simulink model "Problem5"  (R2022a)
settings: Solver=VariableStepAuto  StartTime=0.0  StopTime=t_final  MaxStep=max_step_size  RelTol=1e-3
values from neighbouring files (symbols this model uses):
  k_i_v = k_p_v^2/4    (= 0.25)    [Problem5Part2.m]    (also in Problem5Try1.m; Problem5part15.m; Problem6.m)
  k_p_v = 1    [Problem5Part2.m]    (also in Problem5Try1.m; Problem5part15.m; Problem6.m)
  k_p_y = 4/l_r    (= 2.35294117647)    [Problem5Part2.m]    (also in Problem5Try1.m; Problem5part15.m; Problem6.m)
  l_r = 1.7    [Problem2.m]    (also in Problem2Try2.m; Problem3Try1.m; Problem5Part2.m; Problem5Try1.m)
  psi_initial = psi_sweep(i)    [Problem3Try1.m]    (also in Problem5Part2.m = 0.1; Problem5Try1.m = psi_sweep(j); Problem5part15.m = 0.523598775598; Problem6.m = 0.1)
  v_initial = 0    [Problem5Part2.m]    (also in Problem5Try1.m = v_sweep(i); Problem5part15.m; Problem6.m)
  v_target = 15.6464    [Problem5Part2.m]    (also in Problem5Try1.m; Problem5part15.m; Problem6.m = 20)
  y_initial = 10^(y_sweep(j))    [Problem3Try1.m]    (also in Problem5Part2.m = 0.1; Problem5Try1.m = 10^(log_y_sweep(k)); Problem5part15.m = 0.1; Problem6.m = 0.1)
  y_target = 0    [Problem5Part2.m]    (also in Problem5Try1.m; Problem5part15.m; Problem6.m)
settings Model: Creator=Lawrence  LastModifiedBy=Lawrence

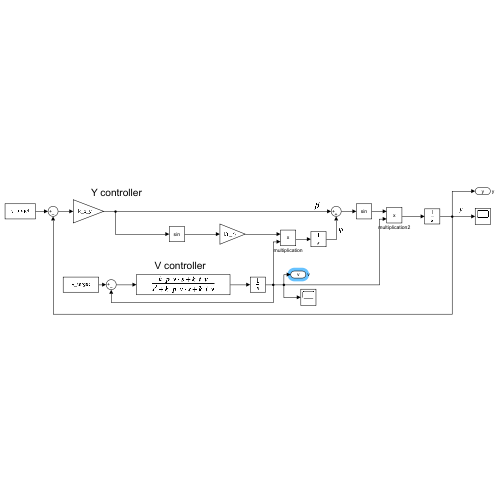
[thumbnail: Simulink's stored preview of the top-level diagram]
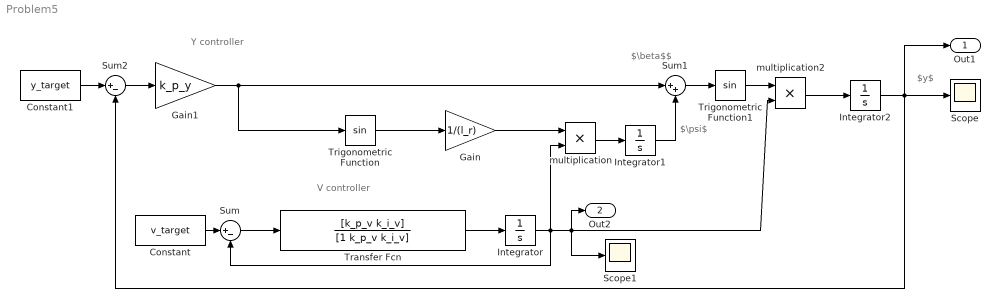
== system Problem5 ==
  note: $y$
  note: $\psi$
  note: $\beta$$
  note: V controller
  note: Y controller
  Constant : Constant  Value=v_target
  Constant1 : Constant  Value=y_target
  Gain : Gain  Gain=1/(l_r)
  Gain1 : Gain  Gain=k_p_y
  Integrator : Integrator  InitialCondition=v_initial
  Integrator1 : Integrator  InitialCondition=psi_initial
  Integrator2 : Integrator  InitialCondition=y_initial
  Scope : Scope
  Scope1 : Scope
  Sum : Sum  Inputs=|+-
  Sum1 : Sum  Inputs=|++
  Sum2 : Sum  Inputs=|+-
  Transfer Fcn : TransferFcn  Numerator=[k_p_v k_i_v]  Denominator=[1 k_p_v k_i_v]
  Trigonometric Function : Trigonometry
  Trigonometric Function1 : Trigonometry
  multiplication : Product
  multiplication2 : Product
  Out1 : Outport  SignalName=y
  Out2 : Outport  Port=2  SignalName=v
  wires:
  Constant/1 -> Sum/1
  Integrator/1 -> Sum/2, Out2/1, Scope1/1, multiplication2/2, multiplication/2
  Trigonometric Function/1 -> Gain/1
  Gain/1 -> multiplication/1
  multiplication/1 -> Integrator1/1
  Gain1/1 -> Sum1/1, Trigonometric Function/1
  Integrator1/1 -> Sum1/2
  Sum1/1 -> Trigonometric Function1/1
  Trigonometric Function1/1 -> multiplication2/1
  multiplication2/1 -> Integrator2/1
  Integrator2/1 -> Out1/1, Scope/1, Sum2/2
  Constant1/1 -> Sum2/1
  Sum2/1 -> Gain1/1
  Sum/1 -> Transfer Fcn/1
  Transfer Fcn/1 -> Integrator/1
